simulink model "sg_2d_fir"  (Simulink 7.6)
settings: Solver=ode45  StartTime=0.0  StopTime=1600.0  RelTol=1e-3
undefined symbols (not defined in the file): gcbh, xlBlockLoadCallback, xlGetNormalizedPeriod, xlipgetpartsetting
libraries: xbsIndex_r4 x311, dspsrcs4 x6
(part 3 of 4)

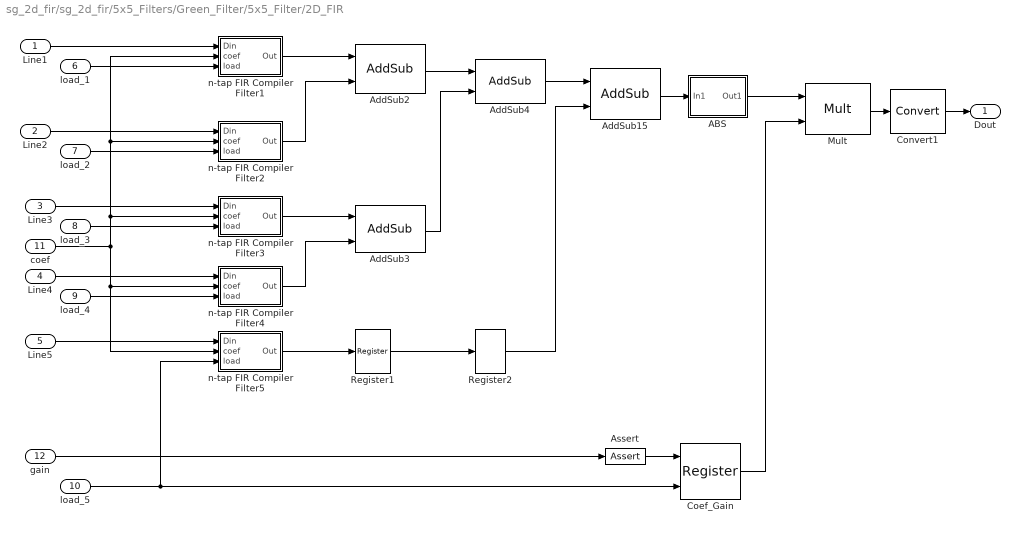
== system sg_2d_fir/sg_2d_fir/5x5_Filters/Green_Filter/5x5_Filter/2D_FIR ==
  Line1 : Inport
  Line2 : Inport  Port=2
  Line3 : Inport  Port=3
  Line4 : Inport  Port=4
  Line5 : Inport  Port=5
  load_1 : Inport  Port=6
  load_2 : Inport  Port=7
  load_3 : Inport  Port=8
  load_4 : Inport  Port=9
  load_5 : Inport  Port=10
  coef : Inport  Port=11
  gain : Inport  Port=12
  ABS : Subsystem
  AddSub{2..4,15} (4 alike) : xbsIndex_r4/AddSub  mode=Addition  use_carryin=off  use_carryout=off  en=off  latency=1  precision=Full  arith_type=Unsigned  n_bits=8  bin_pt=2  quantization=Truncate  overflow=Wrap  dbl_ovrd=off  use_behavioral_HDL=off  hw_selection=Fabric  pipelined=off  use_rpm=off  block_type=addsub
      settings: xl_area=[0, 0, 0, 0, 0, 0, 0]  block_version=VER_STRING_GOES_HERE
  Assert : xbsIndex_r4/Assert  assert_type=on  type_source=Explicitly  gui_display_data_type=Fixed-point  arith_type=Unsigned  n_bits=gain_n_bits  bin_pt=gain_bin_pt  preci_type=Single  exp_width=8  frac_width=24  assert_rate=off  rate_source=Explicitly  period=1  output_port=on  block_type=assert
      settings: infoedit=Asserts a user-defined sample rate and/or type on a signal.<P><P>Hardware notes: In hardware this block costs nothing.  block_version=9.1.01
  Coef_Gain : xbsIndex_r4/Register  init=0  rst=off  en=on  dbl_ovrd=off  block_type=register
      settings: block_version=9.1.01
  Convert1 : xbsIndex_r4/Convert  gui_display_data_type=Fixed-point  arith_type=Unsigned  n_bits=8  bin_pt=0  float_type=Single  exp_bits=8  fraction_bits=24  quantization=Truncate  overflow=Saturate  en=off  latency=1  dbl_ovrd=off  pipeline=off  block_type=convert
      settings: infoedit=The input is presented at the output after quantization and overflow effects.<P><P>Hardware notes: Additional hardware is used when rounding or saturation is selected and output width is less than the input width.  xl_area=[0, 0, 0, 0, 0, 0, 0]  block_version=VER_STRING_GOES_HERE
  Mult : xbsIndex_r4/Mult  precision=Full  arith_type="Signed  (2's comp)"  n_bits=8  bin_pt=2  quantization=Truncate  overflow=Wrap  en=off  latency=4  dbl_ovrd=off  use_behavioral_HDL=off  opt=Speed  use_embedded=on  optimum_pipeline=off  pipeline=off  use_rpm=off  placement_style=Rectangular shape  block_type=mult
      settings: infoedit=Multiplies two values.<P><P>Hardware notes: To use the internal pipeline stage of the dedicated multiplier you must select 'Pipeline to Greatest Extent Possible'.  xl_area=[0, 0, 0, 0, 0, 0, 0]  block_version=VER_STRING_GOES_HERE
  Register1 : xbsIndex_r4/Register  init=0  rst=off  en=off  dbl_ovrd=off  block_type=register
      settings: xl_area=[0, 0, 0, 0, 0, 0, 0]  block_version=VER_STRING_GOES_HERE
  Register2 : xbsIndex_r4/Register  init=0  rst=off  en=off  dbl_ovrd=off  block_type=register
      settings: xl_area=[0, 0, 0, 0, 0, 0, 0]  block_version=VER_STRING_GOES_HERE
  n-tap FIR Compiler Filter1 : Subsystem  mask{coef=maskCoef(1,5:-1:1,maskNum), coef_n_bits=coef_n_bits, coef_bin_pt=coef_bin_pt}
      mask prompts: coef "Coefficients"; coef_n_bits "Number of Bits per Coefficient"; coef_bin_pt "Binary Point for Coefficients"
      mask help: FIR Compiler based FIR filter with n coefficients
      mask init: same as sg_2d_fir/sg_2d_fir/5x5_Filters/Blue_Filter/5x5_Filter/2D_FIR/n-tap FIR Compiler Filter1
      mask Display:
      | patch([0 iWidth iWidth 0],[0 0 iHeight iHeight] , bg);
      | patch(logoX,logoY, fg);
      | text(iCx/1.8,iCy+2,dstr);
      | text(iCx/2.0-4,iCy-10,'FIR Filter');
      | plot([0 0 iWidth iWidth 0], [0 iHeight iHeight 0 0]);
  n-tap FIR Compiler Filter2 : Subsystem  mask{coef=maskCoef(2,5:-1:1,maskNum), coef_n_bits=coef_n_bits, coef_bin_pt=coef_bin_pt}
      mask prompts: coef "Coefficients"; coef_n_bits "Number of Bits per Coefficient"; coef_bin_pt "Binary Point for Coefficients"
      mask help: FIR Compiler based FIR filter with n coefficients
      mask init: same as sg_2d_fir/sg_2d_fir/5x5_Filters/Blue_Filter/5x5_Filter/2D_FIR/n-tap FIR Compiler Filter1
      mask Display:
      | patch([0 iWidth iWidth 0],[0 0 iHeight iHeight] , bg);
      | patch(logoX,logoY, fg);
      | text(iCx/1.8,iCy+2,dstr);
      | text(iCx/2.0-4,iCy-10,'FIR Filter');
      | plot([0 0 iWidth iWidth 0], [0 iHeight iHeight 0 0]);
  n-tap FIR Compiler Filter3 : Subsystem  mask{coef=maskCoef(3,5:-1:1,maskNum), coef_n_bits=coef_n_bits, coef_bin_pt=coef_bin_pt}
      mask prompts: coef "Coefficients"; coef_n_bits "Number of Bits per Coefficient"; coef_bin_pt "Binary Point for Coefficients"
      mask help: FIR Compiler based FIR filter with n coefficients
      mask init: same as sg_2d_fir/sg_2d_fir/5x5_Filters/Blue_Filter/5x5_Filter/2D_FIR/n-tap FIR Compiler Filter1
      mask Display:
      | patch([0 iWidth iWidth 0],[0 0 iHeight iHeight] , bg);
      | patch(logoX,logoY, fg);
      | text(iCx/1.8,iCy+2,dstr);
      | text(iCx/2.0-4,iCy-10,'FIR Filter');
      | plot([0 0 iWidth iWidth 0], [0 iHeight iHeight 0 0]);
  n-tap FIR Compiler Filter4 : Subsystem  mask{coef=maskCoef(4,5:-1:1,maskNum), coef_n_bits=coef_n_bits, coef_bin_pt=coef_bin_pt}
      mask prompts: coef "Coefficients"; coef_n_bits "Number of Bits per Coefficient"; coef_bin_pt "Binary Point for Coefficients"
      mask help: FIR Compiler based FIR filter with n coefficients
      mask init: same as sg_2d_fir/sg_2d_fir/5x5_Filters/Blue_Filter/5x5_Filter/2D_FIR/n-tap FIR Compiler Filter1
      mask Display:
      | patch([0 iWidth iWidth 0],[0 0 iHeight iHeight] , bg);
      | patch(logoX,logoY, fg);
      | text(iCx/1.8,iCy+2,dstr);
      | text(iCx/2.0-4,iCy-10,'FIR Filter');
      | plot([0 0 iWidth iWidth 0], [0 iHeight iHeight 0 0]);
  n-tap FIR Compiler Filter5 : Subsystem  mask{coef=maskCoef(5,5:-1:1,maskNum), coef_n_bits=coef_n_bits, coef_bin_pt=coef_bin_pt}
      mask prompts: coef "Coefficients"; coef_n_bits "Number of Bits per Coefficient"; coef_bin_pt "Binary Point for Coefficients"
      mask help: FIR Compiler based FIR filter with n coefficients
      mask init: same as sg_2d_fir/sg_2d_fir/5x5_Filters/Blue_Filter/5x5_Filter/2D_FIR/n-tap FIR Compiler Filter1
      mask Display:
      | patch([0 iWidth iWidth 0],[0 0 iHeight iHeight] , bg);
      | patch(logoX,logoY, fg);
      | text(iCx/1.8,iCy+2,dstr);
      | text(iCx/2.0-4,iCy-10,'FIR Filter');
      | plot([0 0 iWidth iWidth 0], [0 iHeight iHeight 0 0]);
  Dout : Outport
  wires:
  Assert/1 -> Coef_Gain/1
  coef/1 -> n-tap FIR Compiler Filter5/2(coef), n-tap FIR Compiler Filter4/2(coef), n-tap FIR Compiler Filter3/2(coef), n-tap FIR Compiler Filter2/2(coef), n-tap FIR Compiler Filter1/2(coef)
  load_5/1 -> Coef_Gain/2, n-tap FIR Compiler Filter5/3(load)
  Coef_Gain/1 -> Mult/2
  ABS/1(Out1) -> Mult/1
  Mult/1 -> Convert1/1
  Register2/1 -> AddSub15/2
  AddSub4/1 -> AddSub15/1
  AddSub15/1 -> ABS/1(In1)
  Register1/1 -> Register2/1
  n-tap FIR Compiler Filter5/1(Out) -> Register1/1
  AddSub3/1 -> AddSub4/2
  AddSub2/1 -> AddSub4/1
  n-tap FIR Compiler Filter4/1(Out) -> AddSub3/2
  n-tap FIR Compiler Filter3/1(Out) -> AddSub3/1
  n-tap FIR Compiler Filter2/1(Out) -> AddSub2/2
  n-tap FIR Compiler Filter1/1(Out) -> AddSub2/1
  Line1/1 -> n-tap FIR Compiler Filter1/1(Din)
  load_1/1 -> n-tap FIR Compiler Filter1/3(load)
  Convert1/1 -> Dout/1
  Line2/1 -> n-tap FIR Compiler Filter2/1(Din)
  load_2/1 -> n-tap FIR Compiler Filter2/3(load)
  Line3/1 -> n-tap FIR Compiler Filter3/1(Din)
  load_3/1 -> n-tap FIR Compiler Filter3/3(load)
  Line4/1 -> n-tap FIR Compiler Filter4/1(Din)
  load_4/1 -> n-tap FIR Compiler Filter4/3(load)
  Line5/1 -> n-tap FIR Compiler Filter5/1(Din)
  gain/1 -> Assert/1

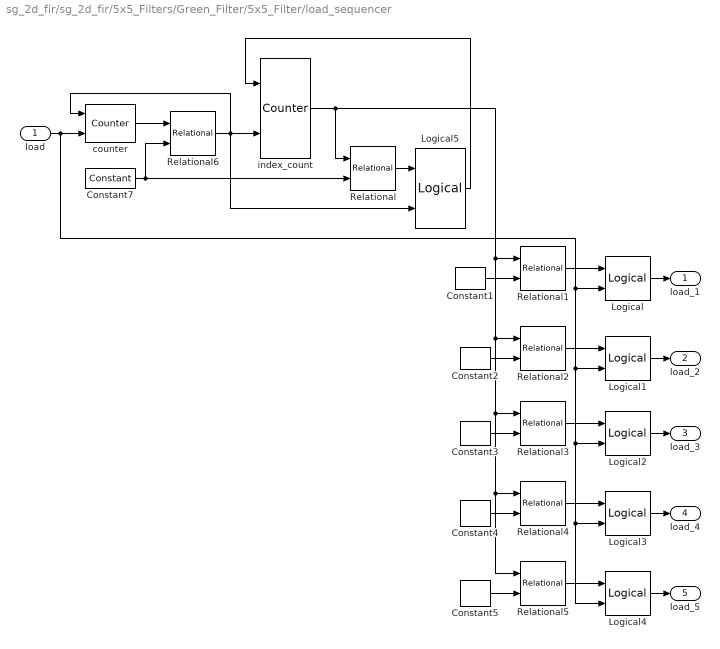
== system sg_2d_fir/sg_2d_fir/5x5_Filters/Green_Filter/5x5_Filter/load_sequencer ==
  load : Inport
  Constant1 : xbsIndex_r4/Constant  const=0  gui_display_data_type=Fixed-point  arith_type=Unsigned  n_bits=ceil(log2(num_coef))  bin_pt=0  preci_type=Single  exp_width=8  frac_width=24  explicit_period=off  period=1  equ=P=C  opselect=C  inp2=PCIN>>17  opr=+  inp1=P  carry=CIN  dbl_ovrd=off  block_type=constant
      settings: block_version=VER_STRING_GOES_HERE
  Constant2 : xbsIndex_r4/Constant  const=1  gui_display_data_type=Fixed-point  arith_type=Unsigned  n_bits=ceil(log2(num_coef))  bin_pt=0  preci_type=Single  exp_width=8  frac_width=24  explicit_period=off  period=1  equ=P=C  opselect=C  inp2=PCIN>>17  opr=+  inp1=P  carry=CIN  dbl_ovrd=off  block_type=constant
      settings: block_version=VER_STRING_GOES_HERE
  Constant3 : xbsIndex_r4/Constant  const=2  gui_display_data_type=Fixed-point  arith_type=Unsigned  n_bits=ceil(log2(num_coef))  bin_pt=0  preci_type=Single  exp_width=8  frac_width=24  explicit_period=off  period=1  equ=P=C  opselect=C  inp2=PCIN>>17  opr=+  inp1=P  carry=CIN  dbl_ovrd=off  block_type=constant
      settings: block_version=VER_STRING_GOES_HERE
  Constant4 : xbsIndex_r4/Constant  const=3  gui_display_data_type=Fixed-point  arith_type=Unsigned  n_bits=ceil(log2(num_coef))  bin_pt=0  preci_type=Single  exp_width=8  frac_width=24  explicit_period=off  period=1  equ=P=C  opselect=C  inp2=PCIN>>17  opr=+  inp1=P  carry=CIN  dbl_ovrd=off  block_type=constant
      settings: block_version=VER_STRING_GOES_HERE
  Constant5 : xbsIndex_r4/Constant  const=4  gui_display_data_type=Fixed-point  arith_type=Unsigned  n_bits=ceil(log2(num_coef))  bin_pt=0  preci_type=Single  exp_width=8  frac_width=24  explicit_period=off  period=1  equ=P=C  opselect=C  inp2=PCIN>>17  opr=+  inp1=P  carry=CIN  dbl_ovrd=off  block_type=constant
      settings: block_version=VER_STRING_GOES_HERE
  Constant7 : xbsIndex_r4/Constant  const=num_coef-1  gui_display_data_type=Fixed-point  arith_type=Unsigned  n_bits=ceil(log2(num_coef))  bin_pt=0  preci_type=Single  exp_width=8  frac_width=24  explicit_period=off  period=1  equ=P=C  opselect=C  inp2=PCIN>>17  opr=+  inp1=P  carry=CIN  dbl_ovrd=off  block_type=constant
      settings: block_version=VER_STRING_GOES_HERE
  Logical{,1..5} (6 alike) : xbsIndex_r4/Logical  logical_function=AND  inputs=2  en=off  latency=0  precision=Full  arith_type=Unsigned  n_bits=8  bin_pt=2  align_bp=on  dbl_ovrd=off  block_type=logical
      settings: xl_area=[0, 0, 0, 0, 0, 0, 0]  block_version=VER_STRING_GOES_HERE
  Relational{,1..6} (7 alike) : xbsIndex_r4/Relational  mode=a=b  en=off  latency=0  dbl_ovrd=off  block_type=relational
      settings: xl_area=[0, 0, 0, 0, 0, 0, 0]  block_version=VER_STRING_GOES_HERE
  counter : xbsIndex_r4/Counter  cnt_type=Count Limited  cnt_to=num_coef-1  operation=Up  start_count=0  cnt_by_val=1  arith_type=Unsigned  n_bits=ceil(log2(num_coef))  bin_pt=0  load_pin=off  rst=on  en=on  explicit_period=on  period=1  dbl_ovrd=off  use_behavioral_HDL=off  implementation=Fabric  use_rpm=off  block_type=counter
      settings: xl_area=[0, 0, 0, 0, 0, 0, 0]  block_version=VER_STRING_GOES_HERE
  index_count : xbsIndex_r4/Counter  cnt_type=Count Limited  cnt_to=num_coef-1  operation=Up  start_count=0  cnt_by_val=1  arith_type=Unsigned  n_bits=ceil(log2(num_coef))  bin_pt=0  load_pin=off  rst=on  en=on  explicit_period=on  period=1  dbl_ovrd=off  use_behavioral_HDL=off  implementation=Fabric  use_rpm=off  block_type=counter
      settings: infoedit="Configurable up, down and up/down counter.<P><P>Hardware notes: Free running counters are the least expensive in hardware.  A count limited counter is implemented by combining a counter with a comparator."  xl_area=[0, 0, 0, 0, 0, 0, 0]  block_version=VER_STRING_GOES_HERE
  load_1 : Outport
  load_2 : Outport  Port=2
  load_3 : Outport  Port=3
  load_4 : Outport  Port=4
  load_5 : Outport  Port=5
  wires:
  Logical5/1 -> index_count/1
  Relational/1 -> Logical5/1
  index_count/1 -> Relational5/1, Relational4/1, Relational3/1, Relational2/1, Relational1/1, Relational/1
  Relational6/1 -> Logical5/2, counter/1, index_count/2
  Constant7/1 -> Relational/2, Relational6/2
  counter/1 -> Relational6/1
  load/1 -> Logical4/2, Logical3/2, Logical2/2, Logical1/2, Logical/2, counter/2
  Relational5/1 -> Logical4/1
  Logical4/1 -> load_5/1
  Constant5/1 -> Relational5/2
  Relational4/1 -> Logical3/1
  Logical3/1 -> load_4/1
  Constant4/1 -> Relational4/2
  Relational3/1 -> Logical2/1
  Logical2/1 -> load_3/1
  Constant3/1 -> Relational3/2
  Relational2/1 -> Logical1/1
  Logical1/1 -> load_2/1
  Constant2/1 -> Relational2/2
  Logical/1 -> load_1/1
  Relational1/1 -> Logical/1
  Constant1/1 -> Relational1/2

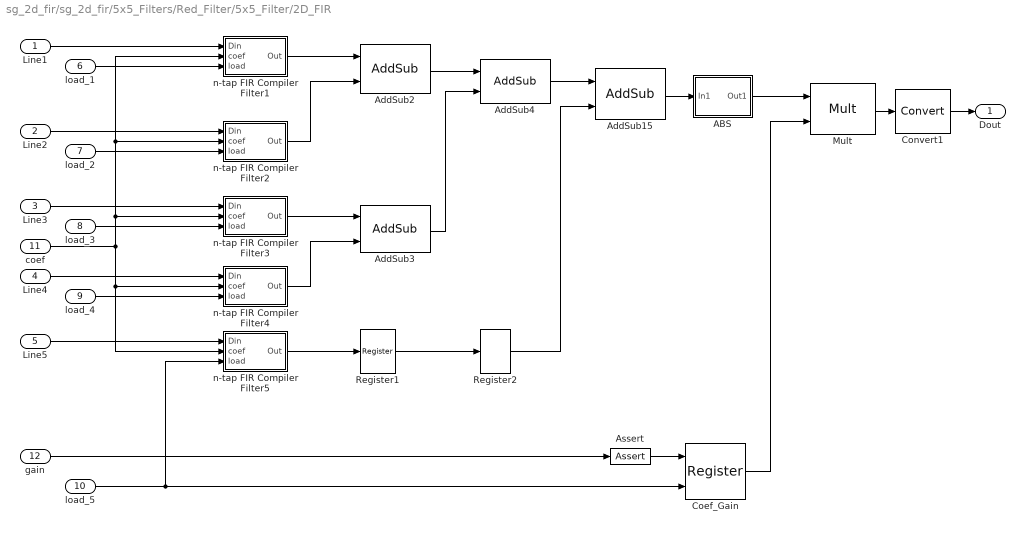
== system sg_2d_fir/sg_2d_fir/5x5_Filters/Red_Filter/5x5_Filter/2D_FIR ==
  Line1 : Inport
  Line2 : Inport  Port=2
  Line3 : Inport  Port=3
  Line4 : Inport  Port=4
  Line5 : Inport  Port=5
  load_1 : Inport  Port=6
  load_2 : Inport  Port=7
  load_3 : Inport  Port=8
  load_4 : Inport  Port=9
  load_5 : Inport  Port=10
  coef : Inport  Port=11
  gain : Inport  Port=12
  ABS : Subsystem
  AddSub{2..4,15} (4 alike) : xbsIndex_r4/AddSub  mode=Addition  use_carryin=off  use_carryout=off  en=off  latency=1  precision=Full  arith_type=Unsigned  n_bits=8  bin_pt=2  quantization=Truncate  overflow=Wrap  dbl_ovrd=off  use_behavioral_HDL=off  hw_selection=Fabric  pipelined=off  use_rpm=off  block_type=addsub
      settings: xl_area=[0, 0, 0, 0, 0, 0, 0]  block_version=VER_STRING_GOES_HERE
  Assert : xbsIndex_r4/Assert  assert_type=on  type_source=Explicitly  gui_display_data_type=Fixed-point  arith_type=Unsigned  n_bits=gain_n_bits  bin_pt=gain_bin_pt  preci_type=Single  exp_width=8  frac_width=24  assert_rate=off  rate_source=Explicitly  period=1  output_port=on  block_type=assert
      settings: infoedit=Asserts a user-defined sample rate and/or type on a signal.<P><P>Hardware notes: In hardware this block costs nothing.  block_version=9.1.01
  Coef_Gain : xbsIndex_r4/Register  init=0  rst=off  en=on  dbl_ovrd=off  block_type=register
      settings: block_version=9.1.01
  Convert1 : xbsIndex_r4/Convert  gui_display_data_type=Fixed-point  arith_type=Unsigned  n_bits=8  bin_pt=0  float_type=Single  exp_bits=8  fraction_bits=24  quantization=Truncate  overflow=Saturate  en=off  latency=1  dbl_ovrd=off  pipeline=off  block_type=convert
      settings: infoedit=The input is presented at the output after quantization and overflow effects.<P><P>Hardware notes: Additional hardware is used when rounding or saturation is selected and output width is less than the input width.  xl_area=[0, 0, 0, 0, 0, 0, 0]  block_version=VER_STRING_GOES_HERE
  Mult : xbsIndex_r4/Mult  precision=Full  arith_type="Signed  (2's comp)"  n_bits=8  bin_pt=2  quantization=Truncate  overflow=Wrap  en=off  latency=4  dbl_ovrd=off  use_behavioral_HDL=off  opt=Speed  use_embedded=on  optimum_pipeline=off  pipeline=off  use_rpm=off  placement_style=Rectangular shape  block_type=mult
      settings: infoedit=Multiplies two values.<P><P>Hardware notes: To use the internal pipeline stage of the dedicated multiplier you must select 'Pipeline to Greatest Extent Possible'.  xl_area=[0, 0, 0, 0, 0, 0, 0]  block_version=VER_STRING_GOES_HERE
  Register1 : xbsIndex_r4/Register  init=0  rst=off  en=off  dbl_ovrd=off  block_type=register
      settings: xl_area=[0, 0, 0, 0, 0, 0, 0]  block_version=VER_STRING_GOES_HERE
  Register2 : xbsIndex_r4/Register  init=0  rst=off  en=off  dbl_ovrd=off  block_type=register
      settings: xl_area=[0, 0, 0, 0, 0, 0, 0]  block_version=VER_STRING_GOES_HERE
  n-tap FIR Compiler Filter1 : Subsystem  mask{coef=maskCoef(1,5:-1:1,maskNum), coef_n_bits=coef_n_bits, coef_bin_pt=coef_bin_pt}
      mask prompts: coef "Coefficients"; coef_n_bits "Number of Bits per Coefficient"; coef_bin_pt "Binary Point for Coefficients"
      mask help: FIR Compiler based FIR filter with n coefficients
      mask init: same as sg_2d_fir/sg_2d_fir/5x5_Filters/Blue_Filter/5x5_Filter/2D_FIR/n-tap FIR Compiler Filter1
      mask Display:
      | patch([0 iWidth iWidth 0],[0 0 iHeight iHeight] , bg);
      | patch(logoX,logoY, fg);
      | text(iCx/1.8,iCy+2,dstr);
      | text(iCx/2.0-4,iCy-10,'FIR Filter');
      | plot([0 0 iWidth iWidth 0], [0 iHeight iHeight 0 0]);
  n-tap FIR Compiler Filter2 : Subsystem  mask{coef=maskCoef(2,5:-1:1,maskNum), coef_n_bits=coef_n_bits, coef_bin_pt=coef_bin_pt}
      mask prompts: coef "Coefficients"; coef_n_bits "Number of Bits per Coefficient"; coef_bin_pt "Binary Point for Coefficients"
      mask help: FIR Compiler based FIR filter with n coefficients
      mask init: same as sg_2d_fir/sg_2d_fir/5x5_Filters/Blue_Filter/5x5_Filter/2D_FIR/n-tap FIR Compiler Filter1
      mask Display:
      | patch([0 iWidth iWidth 0],[0 0 iHeight iHeight] , bg);
      | patch(logoX,logoY, fg);
      | text(iCx/1.8,iCy+2,dstr);
      | text(iCx/2.0-4,iCy-10,'FIR Filter');
      | plot([0 0 iWidth iWidth 0], [0 iHeight iHeight 0 0]);
  n-tap FIR Compiler Filter3 : Subsystem  mask{coef=maskCoef(3,5:-1:1,maskNum), coef_n_bits=coef_n_bits, coef_bin_pt=coef_bin_pt}
      mask prompts: coef "Coefficients"; coef_n_bits "Number of Bits per Coefficient"; coef_bin_pt "Binary Point for Coefficients"
      mask help: FIR Compiler based FIR filter with n coefficients
      mask init: same as sg_2d_fir/sg_2d_fir/5x5_Filters/Blue_Filter/5x5_Filter/2D_FIR/n-tap FIR Compiler Filter1
      mask Display:
      | patch([0 iWidth iWidth 0],[0 0 iHeight iHeight] , bg);
      | patch(logoX,logoY, fg);
      | text(iCx/1.8,iCy+2,dstr);
      | text(iCx/2.0-4,iCy-10,'FIR Filter');
      | plot([0 0 iWidth iWidth 0], [0 iHeight iHeight 0 0]);
  n-tap FIR Compiler Filter4 : Subsystem  mask{coef=maskCoef(4,5:-1:1,maskNum), coef_n_bits=coef_n_bits, coef_bin_pt=coef_bin_pt}
      mask prompts: coef "Coefficients"; coef_n_bits "Number of Bits per Coefficient"; coef_bin_pt "Binary Point for Coefficients"
      mask help: FIR Compiler based FIR filter with n coefficients
      mask init: same as sg_2d_fir/sg_2d_fir/5x5_Filters/Blue_Filter/5x5_Filter/2D_FIR/n-tap FIR Compiler Filter1
      mask Display:
      | patch([0 iWidth iWidth 0],[0 0 iHeight iHeight] , bg);
      | patch(logoX,logoY, fg);
      | text(iCx/1.8,iCy+2,dstr);
      | text(iCx/2.0-4,iCy-10,'FIR Filter');
      | plot([0 0 iWidth iWidth 0], [0 iHeight iHeight 0 0]);
  n-tap FIR Compiler Filter5 : Subsystem  mask{coef=maskCoef(5,5:-1:1,maskNum), coef_n_bits=coef_n_bits, coef_bin_pt=coef_bin_pt}
      mask prompts: coef "Coefficients"; coef_n_bits "Number of Bits per Coefficient"; coef_bin_pt "Binary Point for Coefficients"
      mask help: FIR Compiler based FIR filter with n coefficients
      mask init: same as sg_2d_fir/sg_2d_fir/5x5_Filters/Blue_Filter/5x5_Filter/2D_FIR/n-tap FIR Compiler Filter1
      mask Display:
      | patch([0 iWidth iWidth 0],[0 0 iHeight iHeight] , bg);
      | patch(logoX,logoY, fg);
      | text(iCx/1.8,iCy+2,dstr);
      | text(iCx/2.0-4,iCy-10,'FIR Filter');
      | plot([0 0 iWidth iWidth 0], [0 iHeight iHeight 0 0]);
  Dout : Outport
  wires:
  n-tap FIR Compiler Filter1/1(Out) -> AddSub2/1
  n-tap FIR Compiler Filter2/1(Out) -> AddSub2/2
  n-tap FIR Compiler Filter3/1(Out) -> AddSub3/1
  n-tap FIR Compiler Filter4/1(Out) -> AddSub3/2
  AddSub2/1 -> AddSub4/1
  AddSub3/1 -> AddSub4/2
  n-tap FIR Compiler Filter5/1(Out) -> Register1/1
  Register1/1 -> Register2/1
  AddSub15/1 -> ABS/1(In1)
  AddSub4/1 -> AddSub15/1
  Register2/1 -> AddSub15/2
  Mult/1 -> Convert1/1
  ABS/1(Out1) -> Mult/1
  Coef_Gain/1 -> Mult/2
  load_5/1 -> n-tap FIR Compiler Filter5/3(load), Coef_Gain/2
  coef/1 -> n-tap FIR Compiler Filter1/2(coef), n-tap FIR Compiler Filter2/2(coef), n-tap FIR Compiler Filter3/2(coef), n-tap FIR Compiler Filter4/2(coef), n-tap FIR Compiler Filter5/2(coef)
  Assert/1 -> Coef_Gain/1
  Line1/1 -> n-tap FIR Compiler Filter1/1(Din)
  load_1/1 -> n-tap FIR Compiler Filter1/3(load)
  Convert1/1 -> Dout/1
  Line2/1 -> n-tap FIR Compiler Filter2/1(Din)
  load_2/1 -> n-tap FIR Compiler Filter2/3(load)
  Line3/1 -> n-tap FIR Compiler Filter3/1(Din)
  load_3/1 -> n-tap FIR Compiler Filter3/3(load)
  Line4/1 -> n-tap FIR Compiler Filter4/1(Din)
  load_4/1 -> n-tap FIR Compiler Filter4/3(load)
  Line5/1 -> n-tap FIR Compiler Filter5/1(Din)
  gain/1 -> Assert/1

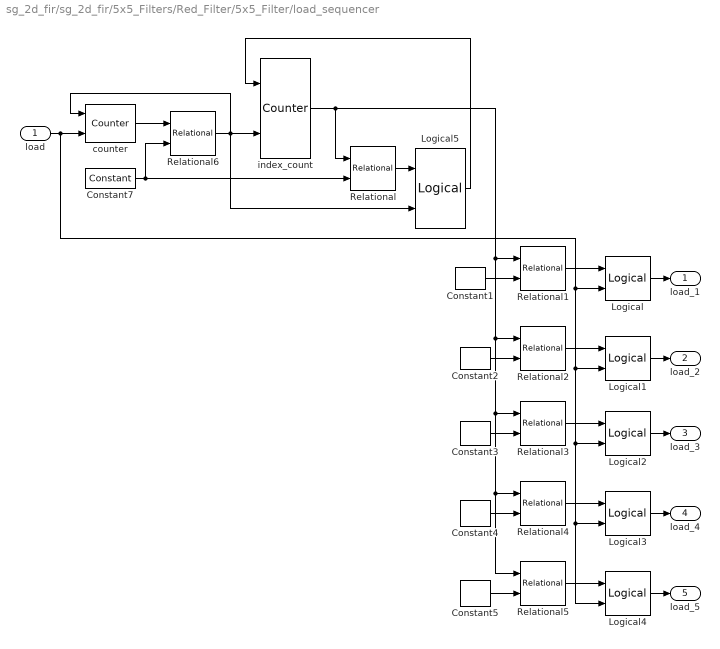
== system sg_2d_fir/sg_2d_fir/5x5_Filters/Red_Filter/5x5_Filter/load_sequencer ==
  load : Inport
  Constant1 : xbsIndex_r4/Constant  const=0  gui_display_data_type=Fixed-point  arith_type=Unsigned  n_bits=ceil(log2(num_coef))  bin_pt=0  preci_type=Single  exp_width=8  frac_width=24  explicit_period=off  period=1  equ=P=C  opselect=C  inp2=PCIN>>17  opr=+  inp1=P  carry=CIN  dbl_ovrd=off  block_type=constant
      settings: block_version=VER_STRING_GOES_HERE
  Constant2 : xbsIndex_r4/Constant  const=1  gui_display_data_type=Fixed-point  arith_type=Unsigned  n_bits=ceil(log2(num_coef))  bin_pt=0  preci_type=Single  exp_width=8  frac_width=24  explicit_period=off  period=1  equ=P=C  opselect=C  inp2=PCIN>>17  opr=+  inp1=P  carry=CIN  dbl_ovrd=off  block_type=constant
      settings: block_version=VER_STRING_GOES_HERE
  Constant3 : xbsIndex_r4/Constant  const=2  gui_display_data_type=Fixed-point  arith_type=Unsigned  n_bits=ceil(log2(num_coef))  bin_pt=0  preci_type=Single  exp_width=8  frac_width=24  explicit_period=off  period=1  equ=P=C  opselect=C  inp2=PCIN>>17  opr=+  inp1=P  carry=CIN  dbl_ovrd=off  block_type=constant
      settings: block_version=VER_STRING_GOES_HERE
  Constant4 : xbsIndex_r4/Constant  const=3  gui_display_data_type=Fixed-point  arith_type=Unsigned  n_bits=ceil(log2(num_coef))  bin_pt=0  preci_type=Single  exp_width=8  frac_width=24  explicit_period=off  period=1  equ=P=C  opselect=C  inp2=PCIN>>17  opr=+  inp1=P  carry=CIN  dbl_ovrd=off  block_type=constant
      settings: block_version=VER_STRING_GOES_HERE
  Constant5 : xbsIndex_r4/Constant  const=4  gui_display_data_type=Fixed-point  arith_type=Unsigned  n_bits=ceil(log2(num_coef))  bin_pt=0  preci_type=Single  exp_width=8  frac_width=24  explicit_period=off  period=1  equ=P=C  opselect=C  inp2=PCIN>>17  opr=+  inp1=P  carry=CIN  dbl_ovrd=off  block_type=constant
      settings: block_version=VER_STRING_GOES_HERE
  Constant7 : xbsIndex_r4/Constant  const=num_coef-1  gui_display_data_type=Fixed-point  arith_type=Unsigned  n_bits=ceil(log2(num_coef))  bin_pt=0  preci_type=Single  exp_width=8  frac_width=24  explicit_period=off  period=1  equ=P=C  opselect=C  inp2=PCIN>>17  opr=+  inp1=P  carry=CIN  dbl_ovrd=off  block_type=constant
      settings: block_version=VER_STRING_GOES_HERE
  Logical{,1..5} (6 alike) : xbsIndex_r4/Logical  logical_function=AND  inputs=2  en=off  latency=0  precision=Full  arith_type=Unsigned  n_bits=8  bin_pt=2  align_bp=on  dbl_ovrd=off  block_type=logical
      settings: xl_area=[0, 0, 0, 0, 0, 0, 0]  block_version=VER_STRING_GOES_HERE
  Relational{,1..6} (7 alike) : xbsIndex_r4/Relational  mode=a=b  en=off  latency=0  dbl_ovrd=off  block_type=relational
      settings: xl_area=[0, 0, 0, 0, 0, 0, 0]  block_version=VER_STRING_GOES_HERE
  counter : xbsIndex_r4/Counter  cnt_type=Count Limited  cnt_to=num_coef-1  operation=Up  start_count=0  cnt_by_val=1  arith_type=Unsigned  n_bits=ceil(log2(num_coef))  bin_pt=0  load_pin=off  rst=on  en=on  explicit_period=on  period=1  dbl_ovrd=off  use_behavioral_HDL=off  implementation=Fabric  use_rpm=off  block_type=counter
      settings: xl_area=[0, 0, 0, 0, 0, 0, 0]  block_version=VER_STRING_GOES_HERE
  index_count : xbsIndex_r4/Counter  cnt_type=Count Limited  cnt_to=num_coef-1  operation=Up  start_count=0  cnt_by_val=1  arith_type=Unsigned  n_bits=ceil(log2(num_coef))  bin_pt=0  load_pin=off  rst=on  en=on  explicit_period=on  period=1  dbl_ovrd=off  use_behavioral_HDL=off  implementation=Fabric  use_rpm=off  block_type=counter
      settings: infoedit="Configurable up, down and up/down counter.<P><P>Hardware notes: Free running counters are the least expensive in hardware.  A count limited counter is implemented by combining a counter with a comparator."  xl_area=[0, 0, 0, 0, 0, 0, 0]  block_version=VER_STRING_GOES_HERE
  load_1 : Outport
  load_2 : Outport  Port=2
  load_3 : Outport  Port=3
  load_4 : Outport  Port=4
  load_5 : Outport  Port=5
  wires:
  Constant1/1 -> Relational1/2
  Relational1/1 -> Logical/1
  Logical/1 -> load_1/1
  Constant2/1 -> Relational2/2
  Logical1/1 -> load_2/1
  Relational2/1 -> Logical1/1
  Constant3/1 -> Relational3/2
  Logical2/1 -> load_3/1
  Relational3/1 -> Logical2/1
  Constant4/1 -> Relational4/2
  Logical3/1 -> load_4/1
  Relational4/1 -> Logical3/1
  Constant5/1 -> Relational5/2
  Logical4/1 -> load_5/1
  Relational5/1 -> Logical4/1
  load/1 -> counter/2, Logical/2, Logical1/2, Logical2/2, Logical3/2, Logical4/2
  counter/1 -> Relational6/1
  Constant7/1 -> Relational6/2, Relational/2
  Relational6/1 -> index_count/2, counter/1, Logical5/2
  index_count/1 -> Relational/1, Relational1/1, Relational2/1, Relational3/1, Relational4/1, Relational5/1
  Relational/1 -> Logical5/1
  Logical5/1 -> index_count/1

== system sg_2d_fir/sg_2d_fir/5x5_Filters/Blue_Filter/5x5_Filter/2D_FIR/ABS ==
  In1 : Inport
  Mux : xbsIndex_r4/Mux  inputs=2  en=off  latency=1  precision=Full  arith_type=Unsigned  n_bits=8  bin_pt=0  quantization=Truncate  overflow=Saturate  dbl_ovrd=off  block_type=mux
      settings: xl_area=[0, 0, 0, 0, 0, 0, 0]  block_version=VER_STRING_GOES_HERE
  Negate : xbsIndex_r4/Negate  precision=Full  arith_type=Unsigned  n_bits=8  bin_pt=2  quantization=Truncate  overflow=Wrap  en=off  latency=1  dbl_ovrd=off  block_type=negate
      settings: xl_area=[0, 0, 0, 0, 0, 0, 0]  block_version=VER_STRING_GOES_HERE
  Register1 : xbsIndex_r4/Register  init=0  rst=off  en=off  dbl_ovrd=off  block_type=register
      settings: xl_area=[0, 0, 0, 0, 0, 0, 0]  block_version=VER_STRING_GOES_HERE
  Register2 : xbsIndex_r4/Register  init=0  rst=off  en=off  dbl_ovrd=off  block_type=register
      settings: xl_area=[0, 0, 0, 0, 0, 0, 0]  block_version=VER_STRING_GOES_HERE
  Slice : xbsIndex_r4/Slice  nbits=1  boolean_output=off  mode=Upper Bit Location + Width  bit1=0  base1=MSB of Input  bit0=0  base0=LSB of Input  dbl_ovrd=off  block_type=slice
      settings: infoedit="Extracts a given range of bits from each input sample and presents it at the output.  The output type is ordinarily unsigned with binary point at zero, but can be Boolean when the slice is one bit wide.<P><P>Hardware notes: In hardware this block costs nothing."  block_version=VER_STRING_GOES_HERE
  Out1 : Outport
  wires:
  Slice/1 -> Register2/1
  Negate/1 -> Mux/3
  In1/1 -> Negate/1, Slice/1, Register1/1
  Mux/1 -> Out1/1
  Register2/1 -> Mux/1
  Register1/1 -> Mux/2

== system sg_2d_fir/sg_2d_fir/5x5_Filters/Blue_Filter/5x5_Filter/2D_FIR/n-tap FIR Compiler Filter1 ==
  Din : Inport
  coef : Inport  Port=2
  load : Inport  Port=3
  "FIR Compiler 5.0 " : xbsIndex_r4/FIR Compiler 5.0   coefficientvector=zeros(1,5)  coefficient_sets=1  filter_type=Single_Rate  rate_change_type=Integer  interpolation_rate=1  decimation_rate=1  zero_pack_factor=1  number_channels=1  ratespecification=Maximum_Possible  sampleperiod=1  hardwareoversamplingrate=1  filter_architecture=Systolic_Multiply_Accumulate  coefficient_reload=on  coefficient_structure=Non_Symmetric  coefficient_sign=Signed  quantization=Quantize_Only  coefficient_width=coef_n_bits  bestprecision=off  coefficient_fractional_bits=coef_bin_pt  number_paths=1  output_rounding_mode=Full_Precision  output_width=26  allow_rounding_approximation=off  optimization_goal=Area  has_sclr=off  has_data_valid=off  has_nd=off  has_ce=off  usechan_in_adv=off  chan_in_adv=0  data_buffer_type=Automatic  coefficient_buffer_type=Automatic  input_buffer_type=Automatic  output_buffer_type=Automatic  preference_for_other_storage=Automatic  multi_column_support=Disabled  columnconfig='1'  inter_column_pipe_length=4  passband_min=0.0  passband_max=0.5  stopband_min=0.5  stopband_max=1.0  filter_selection=1  gui_behaviour=Sysgen  registered_output=true  data_sign=Signed  data_width=16  data_fractional_bits=0  wrapper_available=true  ip_wrap_arbitrary_binary_point=true  ip_name=FIR Compiler  ip_version=5.0  dsptool_ready=true  ipcore_usecache=true  ipcore_useipmodelcache=true  ipcore_xco_need_fpga_part=true  port_translation_map={ 'ce' => 'en', 'sclr' => 'rst' }  run_core_at_system_period=true  ipcore_fpga_part=xlipgetpartsetting(gcb, {'virtex4', 'xc4vsx35', '-10', 'ff668'})  structural_sim=false  block_type=fir_compiler_v5_0
      settings: block_version=11.2
  Register : xbsIndex_r4/Register  init=0  rst=off  en=on  dbl_ovrd=off  block_type=register
  Register2 : xbsIndex_r4/Register  init=0  rst=off  en=off  dbl_ovrd=off  block_type=register
      settings: block_version=9.1-beta
  Rising Edge Detector1 : Subsystem
  Terminator5 : Terminator
  Out : Outport
  wires:
  Din/1 -> "FIR Compiler 5.0 "/1
  "FIR Compiler 5.0 "/3 -> Register/2
  "FIR Compiler 5.0 "/1 -> Register/1
  coef/1 -> "FIR Compiler 5.0 "/4
  Register/1 -> Out/1
  load/1 -> Register2/1, Rising Edge Detector1/1(Din)
  Register2/1 -> "FIR Compiler 5.0 "/3
  Rising Edge Detector1/1(Dout) -> "FIR Compiler 5.0 "/2
  "FIR Compiler 5.0 "/2 -> Terminator5/1

== system sg_2d_fir/sg_2d_fir/5x5_Filters/Blue_Filter/5x5_Filter/2D_FIR/n-tap FIR Compiler Filter2 ==
  Din : Inport
  coef : Inport  Port=2
  load : Inport  Port=3
  "FIR Compiler 5.0 " : xbsIndex_r4/FIR Compiler 5.0   coefficientvector=zeros(1,5)  coefficient_sets=1  filter_type=Single_Rate  rate_change_type=Integer  interpolation_rate=1  decimation_rate=1  zero_pack_factor=1  number_channels=1  ratespecification=Maximum_Possible  sampleperiod=1  hardwareoversamplingrate=1  filter_architecture=Systolic_Multiply_Accumulate  coefficient_reload=on  coefficient_structure=Non_Symmetric  coefficient_sign=Signed  quantization=Quantize_Only  coefficient_width=coef_n_bits  bestprecision=off  coefficient_fractional_bits=coef_bin_pt  number_paths=1  output_rounding_mode=Full_Precision  output_width=26  allow_rounding_approximation=off  optimization_goal=Area  has_sclr=off  has_data_valid=off  has_nd=off  has_ce=off  usechan_in_adv=off  chan_in_adv=0  data_buffer_type=Automatic  coefficient_buffer_type=Automatic  input_buffer_type=Automatic  output_buffer_type=Automatic  preference_for_other_storage=Automatic  multi_column_support=Disabled  columnconfig='1'  inter_column_pipe_length=4  passband_min=0.0  passband_max=0.5  stopband_min=0.5  stopband_max=1.0  filter_selection=1  gui_behaviour=Sysgen  registered_output=true  data_sign=Signed  data_width=16  data_fractional_bits=0  wrapper_available=true  ip_wrap_arbitrary_binary_point=true  ip_name=FIR Compiler  ip_version=5.0  dsptool_ready=true  ipcore_usecache=true  ipcore_useipmodelcache=true  ipcore_xco_need_fpga_part=true  port_translation_map={ 'ce' => 'en', 'sclr' => 'rst' }  run_core_at_system_period=true  ipcore_fpga_part=xlipgetpartsetting(gcb, {'virtex4', 'xc4vsx35', '-10', 'ff668'})  structural_sim=false  block_type=fir_compiler_v5_0
      settings: block_version=11.2
  Register : xbsIndex_r4/Register  init=0  rst=off  en=on  dbl_ovrd=off  block_type=register
  Register2 : xbsIndex_r4/Register  init=0  rst=off  en=off  dbl_ovrd=off  block_type=register
      settings: block_version=9.1-beta
  Rising Edge Detector1 : Subsystem
  Terminator5 : Terminator
  Out : Outport
  wires:
  "FIR Compiler 5.0 "/2 -> Terminator5/1
  Rising Edge Detector1/1(Dout) -> "FIR Compiler 5.0 "/2
  Register2/1 -> "FIR Compiler 5.0 "/3
  load/1 -> Rising Edge Detector1/1(Din), Register2/1
  Register/1 -> Out/1
  coef/1 -> "FIR Compiler 5.0 "/4
  "FIR Compiler 5.0 "/1 -> Register/1
  "FIR Compiler 5.0 "/3 -> Register/2
  Din/1 -> "FIR Compiler 5.0 "/1

== system sg_2d_fir/sg_2d_fir/5x5_Filters/Blue_Filter/5x5_Filter/2D_FIR/n-tap FIR Compiler Filter3 ==
  Din : Inport
  coef : Inport  Port=2
  load : Inport  Port=3
  "FIR Compiler 5.0 " : xbsIndex_r4/FIR Compiler 5.0   coefficientvector=zeros(1,5)  coefficient_sets=1  filter_type=Single_Rate  rate_change_type=Integer  interpolation_rate=1  decimation_rate=1  zero_pack_factor=1  number_channels=1  ratespecification=Maximum_Possible  sampleperiod=1  hardwareoversamplingrate=1  filter_architecture=Systolic_Multiply_Accumulate  coefficient_reload=on  coefficient_structure=Non_Symmetric  coefficient_sign=Signed  quantization=Quantize_Only  coefficient_width=coef_n_bits  bestprecision=off  coefficient_fractional_bits=coef_bin_pt  number_paths=1  output_rounding_mode=Full_Precision  output_width=26  allow_rounding_approximation=off  optimization_goal=Area  has_sclr=off  has_data_valid=off  has_nd=off  has_ce=off  usechan_in_adv=off  chan_in_adv=0  data_buffer_type=Automatic  coefficient_buffer_type=Automatic  input_buffer_type=Automatic  output_buffer_type=Automatic  preference_for_other_storage=Automatic  multi_column_support=Disabled  columnconfig='1'  inter_column_pipe_length=4  passband_min=0.0  passband_max=0.5  stopband_min=0.5  stopband_max=1.0  filter_selection=1  gui_behaviour=Sysgen  registered_output=true  data_sign=Signed  data_width=16  data_fractional_bits=0  wrapper_available=true  ip_wrap_arbitrary_binary_point=true  ip_name=FIR Compiler  ip_version=5.0  dsptool_ready=true  ipcore_usecache=true  ipcore_useipmodelcache=true  ipcore_xco_need_fpga_part=true  port_translation_map={ 'ce' => 'en', 'sclr' => 'rst' }  run_core_at_system_period=true  ipcore_fpga_part=xlipgetpartsetting(gcb, {'virtex4', 'xc4vsx35', '-10', 'ff668'})  structural_sim=false  block_type=fir_compiler_v5_0
      settings: block_version=11.2
  Register : xbsIndex_r4/Register  init=0  rst=off  en=on  dbl_ovrd=off  block_type=register
  Register2 : xbsIndex_r4/Register  init=0  rst=off  en=off  dbl_ovrd=off  block_type=register
      settings: block_version=9.1-beta
  Rising Edge Detector1 : Subsystem
  Terminator5 : Terminator
  Out : Outport
  wires:
  Din/1 -> "FIR Compiler 5.0 "/1
  "FIR Compiler 5.0 "/3 -> Register/2
  "FIR Compiler 5.0 "/1 -> Register/1
  coef/1 -> "FIR Compiler 5.0 "/4
  Register/1 -> Out/1
  load/1 -> Register2/1, Rising Edge Detector1/1(Din)
  Register2/1 -> "FIR Compiler 5.0 "/3
  Rising Edge Detector1/1(Dout) -> "FIR Compiler 5.0 "/2
  "FIR Compiler 5.0 "/2 -> Terminator5/1

== system sg_2d_fir/sg_2d_fir/5x5_Filters/Blue_Filter/5x5_Filter/2D_FIR/n-tap FIR Compiler Filter4 ==
  Din : Inport
  coef : Inport  Port=2
  load : Inport  Port=3
  "FIR Compiler 5.0 " : xbsIndex_r4/FIR Compiler 5.0   coefficientvector=zeros(1,5)  coefficient_sets=1  filter_type=Single_Rate  rate_change_type=Integer  interpolation_rate=1  decimation_rate=1  zero_pack_factor=1  number_channels=1  ratespecification=Maximum_Possible  sampleperiod=1  hardwareoversamplingrate=1  filter_architecture=Systolic_Multiply_Accumulate  coefficient_reload=on  coefficient_structure=Non_Symmetric  coefficient_sign=Signed  quantization=Quantize_Only  coefficient_width=coef_n_bits  bestprecision=off  coefficient_fractional_bits=coef_bin_pt  number_paths=1  output_rounding_mode=Full_Precision  output_width=26  allow_rounding_approximation=off  optimization_goal=Area  has_sclr=off  has_data_valid=off  has_nd=off  has_ce=off  usechan_in_adv=off  chan_in_adv=0  data_buffer_type=Automatic  coefficient_buffer_type=Automatic  input_buffer_type=Automatic  output_buffer_type=Automatic  preference_for_other_storage=Automatic  multi_column_support=Disabled  columnconfig='1'  inter_column_pipe_length=4  passband_min=0.0  passband_max=0.5  stopband_min=0.5  stopband_max=1.0  filter_selection=1  gui_behaviour=Sysgen  registered_output=true  data_sign=Signed  data_width=16  data_fractional_bits=0  wrapper_available=true  ip_wrap_arbitrary_binary_point=true  ip_name=FIR Compiler  ip_version=5.0  dsptool_ready=true  ipcore_usecache=true  ipcore_useipmodelcache=true  ipcore_xco_need_fpga_part=true  port_translation_map={ 'ce' => 'en', 'sclr' => 'rst' }  run_core_at_system_period=true  ipcore_fpga_part=xlipgetpartsetting(gcb, {'virtex4', 'xc4vsx35', '-10', 'ff668'})  structural_sim=false  block_type=fir_compiler_v5_0
      settings: block_version=11.2
  Register : xbsIndex_r4/Register  init=0  rst=off  en=on  dbl_ovrd=off  block_type=register
  Register2 : xbsIndex_r4/Register  init=0  rst=off  en=off  dbl_ovrd=off  block_type=register
      settings: block_version=9.1-beta
  Rising Edge Detector1 : Subsystem
  Terminator5 : Terminator
  Out : Outport
  wires:
  "FIR Compiler 5.0 "/2 -> Terminator5/1
  Rising Edge Detector1/1(Dout) -> "FIR Compiler 5.0 "/2
  Register2/1 -> "FIR Compiler 5.0 "/3
  load/1 -> Rising Edge Detector1/1(Din), Register2/1
  Register/1 -> Out/1
  coef/1 -> "FIR Compiler 5.0 "/4
  "FIR Compiler 5.0 "/1 -> Register/1
  "FIR Compiler 5.0 "/3 -> Register/2
  Din/1 -> "FIR Compiler 5.0 "/1

== system sg_2d_fir/sg_2d_fir/5x5_Filters/Blue_Filter/5x5_Filter/2D_FIR/n-tap FIR Compiler Filter5 ==
  Din : Inport
  coef : Inport  Port=2
  load : Inport  Port=3
  "FIR Compiler 5.0 " : xbsIndex_r4/FIR Compiler 5.0   coefficientvector=zeros(1,5)  coefficient_sets=1  filter_type=Single_Rate  rate_change_type=Integer  interpolation_rate=1  decimation_rate=1  zero_pack_factor=1  number_channels=1  ratespecification=Maximum_Possible  sampleperiod=1  hardwareoversamplingrate=1  filter_architecture=Systolic_Multiply_Accumulate  coefficient_reload=on  coefficient_structure=Non_Symmetric  coefficient_sign=Signed  quantization=Quantize_Only  coefficient_width=coef_n_bits  bestprecision=off  coefficient_fractional_bits=coef_bin_pt  number_paths=1  output_rounding_mode=Full_Precision  output_width=26  allow_rounding_approximation=off  optimization_goal=Area  has_sclr=off  has_data_valid=off  has_nd=off  has_ce=off  usechan_in_adv=off  chan_in_adv=0  data_buffer_type=Automatic  coefficient_buffer_type=Automatic  input_buffer_type=Automatic  output_buffer_type=Automatic  preference_for_other_storage=Automatic  multi_column_support=Disabled  columnconfig='1'  inter_column_pipe_length=4  passband_min=0.0  passband_max=0.5  stopband_min=0.5  stopband_max=1.0  filter_selection=1  gui_behaviour=Sysgen  registered_output=true  data_sign=Signed  data_width=16  data_fractional_bits=0  wrapper_available=true  ip_wrap_arbitrary_binary_point=true  ip_name=FIR Compiler  ip_version=5.0  dsptool_ready=true  ipcore_usecache=true  ipcore_useipmodelcache=true  ipcore_xco_need_fpga_part=true  port_translation_map={ 'ce' => 'en', 'sclr' => 'rst' }  run_core_at_system_period=true  ipcore_fpga_part=xlipgetpartsetting(gcb, {'virtex4', 'xc4vsx35', '-10', 'ff668'})  structural_sim=false  block_type=fir_compiler_v5_0
      settings: block_version=11.2
  Register : xbsIndex_r4/Register  init=0  rst=off  en=on  dbl_ovrd=off  block_type=register
  Register2 : xbsIndex_r4/Register  init=0  rst=off  en=off  dbl_ovrd=off  block_type=register
      settings: block_version=9.1-beta
  Rising Edge Detector1 : Subsystem
  Terminator5 : Terminator
  Out : Outport
  wires:
  Din/1 -> "FIR Compiler 5.0 "/1
  "FIR Compiler 5.0 "/3 -> Register/2
  "FIR Compiler 5.0 "/1 -> Register/1
  coef/1 -> "FIR Compiler 5.0 "/4
  Register/1 -> Out/1
  load/1 -> Register2/1, Rising Edge Detector1/1(Din)
  Register2/1 -> "FIR Compiler 5.0 "/3
  Rising Edge Detector1/1(Dout) -> "FIR Compiler 5.0 "/2
  "FIR Compiler 5.0 "/2 -> Terminator5/1

== system sg_2d_fir/sg_2d_fir/5x5_Filters/Green_Filter/5x5_Filter/2D_FIR/ABS ==
  In1 : Inport
  Mux : xbsIndex_r4/Mux  inputs=2  en=off  latency=1  precision=Full  arith_type=Unsigned  n_bits=8  bin_pt=0  quantization=Truncate  overflow=Saturate  dbl_ovrd=off  block_type=mux
      settings: xl_area=[0, 0, 0, 0, 0, 0, 0]  block_version=VER_STRING_GOES_HERE
  Negate : xbsIndex_r4/Negate  precision=Full  arith_type=Unsigned  n_bits=8  bin_pt=2  quantization=Truncate  overflow=Wrap  en=off  latency=1  dbl_ovrd=off  block_type=negate
      settings: xl_area=[0, 0, 0, 0, 0, 0, 0]  block_version=VER_STRING_GOES_HERE
  Register1 : xbsIndex_r4/Register  init=0  rst=off  en=off  dbl_ovrd=off  block_type=register
      settings: xl_area=[0, 0, 0, 0, 0, 0, 0]  block_version=VER_STRING_GOES_HERE
  Register2 : xbsIndex_r4/Register  init=0  rst=off  en=off  dbl_ovrd=off  block_type=register
      settings: xl_area=[0, 0, 0, 0, 0, 0, 0]  block_version=VER_STRING_GOES_HERE
  Slice : xbsIndex_r4/Slice  nbits=1  boolean_output=off  mode=Upper Bit Location + Width  bit1=0  base1=MSB of Input  bit0=0  base0=LSB of Input  dbl_ovrd=off  block_type=slice
      settings: infoedit="Extracts a given range of bits from each input sample and presents it at the output.  The output type is ordinarily unsigned with binary point at zero, but can be Boolean when the slice is one bit wide.<P><P>Hardware notes: In hardware this block costs nothing."  block_version=VER_STRING_GOES_HERE
  Out1 : Outport
  wires:
  Slice/1 -> Register2/1
  Negate/1 -> Mux/3
  In1/1 -> Negate/1, Slice/1, Register1/1
  Mux/1 -> Out1/1
  Register2/1 -> Mux/1
  Register1/1 -> Mux/2

== system sg_2d_fir/sg_2d_fir/5x5_Filters/Green_Filter/5x5_Filter/2D_FIR/n-tap FIR Compiler Filter1 ==
  Din : Inport
  coef : Inport  Port=2
  load : Inport  Port=3
  "FIR Compiler 5.0 " : xbsIndex_r4/FIR Compiler 5.0   coefficientvector=zeros(1,5)  coefficient_sets=1  filter_type=Single_Rate  rate_change_type=Integer  interpolation_rate=1  decimation_rate=1  zero_pack_factor=1  number_channels=1  ratespecification=Maximum_Possible  sampleperiod=1  hardwareoversamplingrate=1  filter_architecture=Systolic_Multiply_Accumulate  coefficient_reload=on  coefficient_structure=Non_Symmetric  coefficient_sign=Signed  quantization=Quantize_Only  coefficient_width=coef_n_bits  bestprecision=off  coefficient_fractional_bits=coef_bin_pt  number_paths=1  output_rounding_mode=Full_Precision  output_width=26  allow_rounding_approximation=off  optimization_goal=Area  has_sclr=off  has_data_valid=off  has_nd=off  has_ce=off  usechan_in_adv=off  chan_in_adv=0  data_buffer_type=Automatic  coefficient_buffer_type=Automatic  input_buffer_type=Automatic  output_buffer_type=Automatic  preference_for_other_storage=Automatic  multi_column_support=Disabled  columnconfig='1'  inter_column_pipe_length=4  passband_min=0.0  passband_max=0.5  stopband_min=0.5  stopband_max=1.0  filter_selection=1  gui_behaviour=Sysgen  registered_output=true  data_sign=Signed  data_width=16  data_fractional_bits=0  wrapper_available=true  ip_wrap_arbitrary_binary_point=true  ip_name=FIR Compiler  ip_version=5.0  dsptool_ready=true  ipcore_usecache=true  ipcore_useipmodelcache=true  ipcore_xco_need_fpga_part=true  port_translation_map={ 'ce' => 'en', 'sclr' => 'rst' }  run_core_at_system_period=true  ipcore_fpga_part=xlipgetpartsetting(gcb, {'virtex4', 'xc4vsx35', '-10', 'ff668'})  structural_sim=false  block_type=fir_compiler_v5_0
      settings: block_version=11.2
  Register : xbsIndex_r4/Register  init=0  rst=off  en=on  dbl_ovrd=off  block_type=register
  Register2 : xbsIndex_r4/Register  init=0  rst=off  en=off  dbl_ovrd=off  block_type=register
      settings: block_version=9.1-beta
  Rising Edge Detector1 : Subsystem
  Terminator5 : Terminator
  Out : Outport
  wires:
  Din/1 -> "FIR Compiler 5.0 "/1
  "FIR Compiler 5.0 "/3 -> Register/2
  "FIR Compiler 5.0 "/1 -> Register/1
  coef/1 -> "FIR Compiler 5.0 "/4
  Register/1 -> Out/1
  load/1 -> Register2/1, Rising Edge Detector1/1(Din)
  Register2/1 -> "FIR Compiler 5.0 "/3
  Rising Edge Detector1/1(Dout) -> "FIR Compiler 5.0 "/2
  "FIR Compiler 5.0 "/2 -> Terminator5/1

== system sg_2d_fir/sg_2d_fir/5x5_Filters/Green_Filter/5x5_Filter/2D_FIR/n-tap FIR Compiler Filter2 ==
  Din : Inport
  coef : Inport  Port=2
  load : Inport  Port=3
  "FIR Compiler 5.0 " : xbsIndex_r4/FIR Compiler 5.0   coefficientvector=zeros(1,5)  coefficient_sets=1  filter_type=Single_Rate  rate_change_type=Integer  interpolation_rate=1  decimation_rate=1  zero_pack_factor=1  number_channels=1  ratespecification=Maximum_Possible  sampleperiod=1  hardwareoversamplingrate=1  filter_architecture=Systolic_Multiply_Accumulate  coefficient_reload=on  coefficient_structure=Non_Symmetric  coefficient_sign=Signed  quantization=Quantize_Only  coefficient_width=coef_n_bits  bestprecision=off  coefficient_fractional_bits=coef_bin_pt  number_paths=1  output_rounding_mode=Full_Precision  output_width=26  allow_rounding_approximation=off  optimization_goal=Area  has_sclr=off  has_data_valid=off  has_nd=off  has_ce=off  usechan_in_adv=off  chan_in_adv=0  data_buffer_type=Automatic  coefficient_buffer_type=Automatic  input_buffer_type=Automatic  output_buffer_type=Automatic  preference_for_other_storage=Automatic  multi_column_support=Disabled  columnconfig='1'  inter_column_pipe_length=4  passband_min=0.0  passband_max=0.5  stopband_min=0.5  stopband_max=1.0  filter_selection=1  gui_behaviour=Sysgen  registered_output=true  data_sign=Signed  data_width=16  data_fractional_bits=0  wrapper_available=true  ip_wrap_arbitrary_binary_point=true  ip_name=FIR Compiler  ip_version=5.0  dsptool_ready=true  ipcore_usecache=true  ipcore_useipmodelcache=true  ipcore_xco_need_fpga_part=true  port_translation_map={ 'ce' => 'en', 'sclr' => 'rst' }  run_core_at_system_period=true  ipcore_fpga_part=xlipgetpartsetting(gcb, {'virtex4', 'xc4vsx35', '-10', 'ff668'})  structural_sim=false  block_type=fir_compiler_v5_0
      settings: block_version=11.2
  Register : xbsIndex_r4/Register  init=0  rst=off  en=on  dbl_ovrd=off  block_type=register
  Register2 : xbsIndex_r4/Register  init=0  rst=off  en=off  dbl_ovrd=off  block_type=register
      settings: block_version=9.1-beta
  Rising Edge Detector1 : Subsystem
  Terminator5 : Terminator
  Out : Outport
  wires:
  "FIR Compiler 5.0 "/2 -> Terminator5/1
  Rising Edge Detector1/1(Dout) -> "FIR Compiler 5.0 "/2
  Register2/1 -> "FIR Compiler 5.0 "/3
  load/1 -> Rising Edge Detector1/1(Din), Register2/1
  Register/1 -> Out/1
  coef/1 -> "FIR Compiler 5.0 "/4
  "FIR Compiler 5.0 "/1 -> Register/1
  "FIR Compiler 5.0 "/3 -> Register/2
  Din/1 -> "FIR Compiler 5.0 "/1

== system sg_2d_fir/sg_2d_fir/5x5_Filters/Green_Filter/5x5_Filter/2D_FIR/n-tap FIR Compiler Filter3 ==
  Din : Inport
  coef : Inport  Port=2
  load : Inport  Port=3
  "FIR Compiler 5.0 " : xbsIndex_r4/FIR Compiler 5.0   coefficientvector=zeros(1,5)  coefficient_sets=1  filter_type=Single_Rate  rate_change_type=Integer  interpolation_rate=1  decimation_rate=1  zero_pack_factor=1  number_channels=1  ratespecification=Maximum_Possible  sampleperiod=1  hardwareoversamplingrate=1  filter_architecture=Systolic_Multiply_Accumulate  coefficient_reload=on  coefficient_structure=Non_Symmetric  coefficient_sign=Signed  quantization=Quantize_Only  coefficient_width=coef_n_bits  bestprecision=off  coefficient_fractional_bits=coef_bin_pt  number_paths=1  output_rounding_mode=Full_Precision  output_width=26  allow_rounding_approximation=off  optimization_goal=Area  has_sclr=off  has_data_valid=off  has_nd=off  has_ce=off  usechan_in_adv=off  chan_in_adv=0  data_buffer_type=Automatic  coefficient_buffer_type=Automatic  input_buffer_type=Automatic  output_buffer_type=Automatic  preference_for_other_storage=Automatic  multi_column_support=Disabled  columnconfig='1'  inter_column_pipe_length=4  passband_min=0.0  passband_max=0.5  stopband_min=0.5  stopband_max=1.0  filter_selection=1  gui_behaviour=Sysgen  registered_output=true  data_sign=Signed  data_width=16  data_fractional_bits=0  wrapper_available=true  ip_wrap_arbitrary_binary_point=true  ip_name=FIR Compiler  ip_version=5.0  dsptool_ready=true  ipcore_usecache=true  ipcore_useipmodelcache=true  ipcore_xco_need_fpga_part=true  port_translation_map={ 'ce' => 'en', 'sclr' => 'rst' }  run_core_at_system_period=true  ipcore_fpga_part=xlipgetpartsetting(gcb, {'virtex4', 'xc4vsx35', '-10', 'ff668'})  structural_sim=false  block_type=fir_compiler_v5_0
      settings: block_version=11.2
  Register : xbsIndex_r4/Register  init=0  rst=off  en=on  dbl_ovrd=off  block_type=register
  Register2 : xbsIndex_r4/Register  init=0  rst=off  en=off  dbl_ovrd=off  block_type=register
      settings: block_version=9.1-beta
  Rising Edge Detector1 : Subsystem
  Terminator5 : Terminator
  Out : Outport
  wires:
  Din/1 -> "FIR Compiler 5.0 "/1
  "FIR Compiler 5.0 "/3 -> Register/2
  "FIR Compiler 5.0 "/1 -> Register/1
  coef/1 -> "FIR Compiler 5.0 "/4
  Register/1 -> Out/1
  load/1 -> Register2/1, Rising Edge Detector1/1(Din)
  Register2/1 -> "FIR Compiler 5.0 "/3
  Rising Edge Detector1/1(Dout) -> "FIR Compiler 5.0 "/2
  "FIR Compiler 5.0 "/2 -> Terminator5/1
